simulink model "rsgTask_Complete_t5_bld"  (R2012b)
settings: Solver=FixedStepDiscrete  StartTime=0.0  StopTime=inf  FixedStep=0.001  RelTol=1e-3
settings Model: ExplicitPartitioning=on  Creator=gilja  LastModifiedBy=NPTL
settings SolverCC: EnableConcurrentExecution=on  ConcurrentTasks=on
settings OptimizationCC: InlineParams=on  InlineInvariantSignals=on  EnhancedBackFolding=on  EfficientFloat2IntCast=on
settings HardwareCC: ProdIntDivRoundTo=Zero  ProdEndianess=LittleEndian  ProdHWDeviceType=Generic->32-bit x86 compatible
settings ModelReferenceCC: UpdateModelReferenceTargets=IfOutOfDate  ModelReferenceMinAlgLoopOccurrences=on
settings RTWCC: SystemTargetFile=xpctarget.tlc  TLCOptions=-axPCMaxOverloads=10000 -axPCOverLoadLen=5 -axPCStartupFlag=200  TemplateMakefile=xpc_default_tmf  Description=xPC Target  ProcessScript=xpctarget_make_rtw_hook  RTWUseSimCustomCode=on  RTWCompilerOptimization=On
settings CodeAppCC: MaxIdLength=62
settings xpcTargetCC: TargetFcnLib=ansi_tfl_table_tmw.mat  CodeReplacementLibrary=XPC_BLAS  ParMdlRefBuildCompliant=on  ConcurrentExecutionCompliant=on  CombineSignalStateStructs=off  GRTInterface=on  xPCTaskExecutionProfile=on  xPCRL32EventNumber=5000  RL32IRQSourceModifier=5  xPCIRQSourceBoard=Parallel_Port  xPCIOIRQSlot=0x378  xPCisDownloadable=off  xPCLoadParamSetFile=off  xPCConcurrentTasks=off  xPCEnableSFAnimation=off

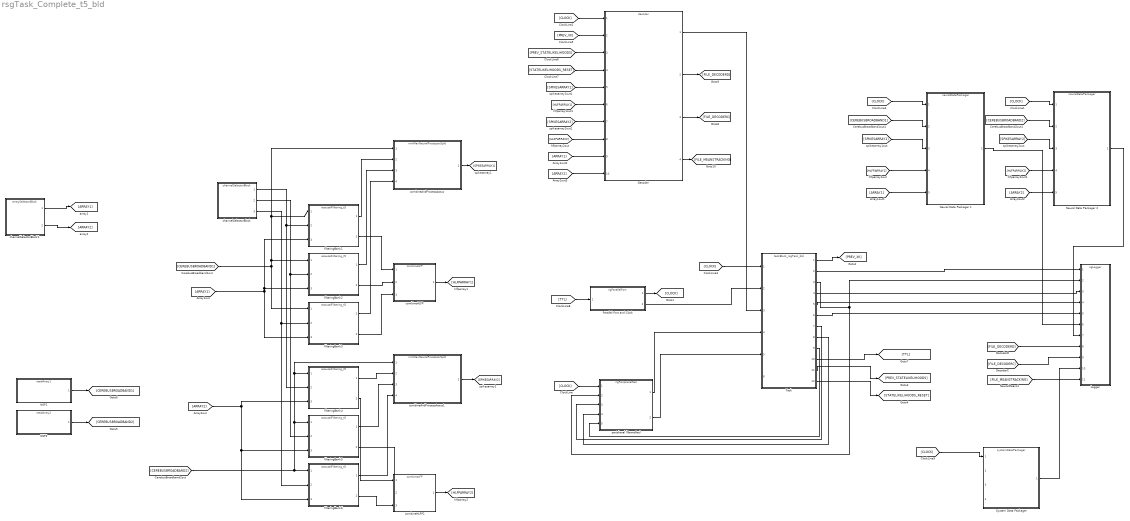
== system rsgTask_Complete_t5_bld ==
  Decoder : ModelReference  ModelNameDialog=decoder  SimulationMode=Normal  ModelReferenceVersion=1.1425  CopyOfModelName=decoder  DefaultDataLogging=on
  Logger : ModelReference  ModelNameDialog=rigLogger  SimulationMode=Normal  ModelReferenceVersion=1.138  CopyOfModelName=rigLogger  DefaultDataLogging=on
  NSP1 : ModelReference  ModelNameDialog=readArray1  SimulationMode=Normal  ModelReferenceVersion=1.166  CopyOfModelName=readArray1  DefaultDataLogging=on
  NSP2 : ModelReference  ModelNameDialog=readArray2  SimulationMode=Normal  ModelReferenceVersion=1.127  CopyOfModelName=readArray2  DefaultDataLogging=on
  Neural Data Packager 1 : ModelReference  ModelNameDialog=neuralDataPackager  SimulationMode=Normal  ModelReferenceVersion=1.174  CopyOfModelName=neuralDataPackager  DefaultDataLogging=on
  Neural Data Packager 2 : ModelReference  ModelNameDialog=neuralDataPackager  SimulationMode=Normal  ModelReferenceVersion=1.174  CopyOfModelName=neuralDataPackager  DefaultDataLogging=on
  Parallel Port and Clock : ModelReference  ModelNameDialog=rigParallelPort  SimulationMode=Normal  ModelReferenceVersion=1.93  CopyOfModelName=rigParallelPort  DefaultDataLogging=on
  System Data Packager : ModelReference  Priority=0  ModelNameDialog=systemDataPackager  SimulationMode=Normal  ModelReferenceVersion=1.180  CopyOfModelName=systemDataPackager  DefaultDataLogging=on
  Task : ModelReference  ModelNameDialog=taskBlock_rsgTask_bld  SimulationMode=Normal  ModelReferenceVersion=1.983  CopyOfModelName=taskBlock_rsgTask_bld  DefaultDataLogging=on
  channelSelectorBlock : ModelReference  ModelNameDialog=channelSelectorBlock  SimulationMode=Normal  ModelReferenceVersion=1.36  CopyOfModelName=channelSelectorBlock  DefaultDataLogging=on
  channelSelectorBlock1 : ModelReference  ModelNameDialog=arraySelectorBlock  SimulationMode=Normal  ModelReferenceVersion=1.40  CopyOfModelName=arraySelectorBlock  DefaultDataLogging=on
  combineAndProcessAcaus : ModelReference  ModelNameDialog=minMaxNeuralProcessorSplit  SimulationMode=Normal  ModelReferenceVersion=1.38  CopyOfModelName=minMaxNeuralProcessorSplit  DefaultDataLogging=on
  combineAndProcessAcaus1 : ModelReference  ModelNameDialog=minMaxNeuralProcessorSplit  SimulationMode=Normal  ModelReferenceVersion=1.38  CopyOfModelName=minMaxNeuralProcessorSplit  DefaultDataLogging=on
  combineHLFP : ModelReference  ModelNameDialog=combineLFP  SimulationMode=Normal  ModelReferenceVersion=1.38  CopyOfModelName=combineLFP  DefaultDataLogging=on
  combineHLFP1 : ModelReference  ModelNameDialog=combineLFP  SimulationMode=Normal  ModelReferenceVersion=1.38  CopyOfModelName=combineLFP  DefaultDataLogging=on
  filteringBank{1..6} (6 alike) : ModelReference  ModelNameDialog=acausalFiltering_t5  SimulationMode=Normal  ModelReferenceVersion=1.78  CopyOfModelName=acausalFiltering_t5  DefaultDataLogging=on
  peripheral (GameNet) : ModelReference  ModelNameDialog=rigPeripheralNet  SimulationMode=Normal  ModelReferenceVersion=1.372  CopyOfModelName=rigPeripheralNet  DefaultDataLogging=on
  wires:
  filteringBank1/1 -> combineAndProcessAcaus/2
  channelSelectorBlock/1 -> filteringBank4/2, filteringBank1/2
  channelSelectorBlock/2 -> filteringBank5/2, filteringBank2/2
  filteringBank2/1 -> combineAndProcessAcaus/3
  channelSelectorBlock/3 -> filteringBank6/2, filteringBank3/2
  filteringBank3/1 -> combineAndProcessAcaus/4
  filteringBank1/2 -> combineHLFP/1
  filteringBank2/2 -> combineHLFP/2
  filteringBank3/2 -> combineHLFP/3
  Parallel Port and Clock/2 -> Task/2
  [SPIKESARRAY1] -> Neural Data Packager 1/3
  Decoder/1 -> Task/3
  Neural Data Packager 1/1 -> Logger/6
  Task/2 -> Logger/1
  Task/3 -> peripheral (GameNet)/2, Logger/2
  Task/4 -> Logger/3
  Task/5 -> Logger/4
  Task/6 -> Logger/5
  Task/7 -> peripheral (GameNet)/3
  peripheral (GameNet)/1 -> Task/4
  peripheral (GameNet)/2 -> Task/5
  Task/9 -> peripheral (GameNet)/5
  Task/8 -> peripheral (GameNet)/4
  [CEREBUSBROADBAND1] -> filteringBank3/1, filteringBank2/1, combineAndProcessAcaus/1, filteringBank1/1
  [CEREBUSBROADBAND2] -> filteringBank6/1, filteringBank5/1, filteringBank4/1, combineAndProcessAcaus1/1
  filteringBank5/2 -> combineHLFP1/2
  filteringBank4/2 -> combineHLFP1/1
  filteringBank6/2 -> combineHLFP1/3
  filteringBank4/1 -> combineAndProcessAcaus1/2
  filteringBank5/1 -> combineAndProcessAcaus1/3
  filteringBank6/1 -> combineAndProcessAcaus1/4
  Neural Data Packager 2/1 -> Logger/7
  [ARRAY1] -> filteringBank3/3, filteringBank1/3, filteringBank2/3
  [ARRAY2] -> filteringBank4/3, filteringBank6/3, filteringBank5/3
  Parallel Port and Clock/1 -> [CLOCK]
  [CLOCK] -> peripheral (GameNet)/1
  [CLOCK] -> Neural Data Packager 2/1
  [CLOCK] -> Decoder/1
  [CLOCK] -> Task/1
  [CLOCK] -> Neural Data Packager 1/1
  combineHLFP/1 -> [HLFPARRAY1]
  [HLFPARRAY1] -> Neural Data Packager 1/4
  [HLFPARRAY1] -> Decoder/6
  combineHLFP1/1 -> [HLFPARRAY2]
  [HLFPARRAY2] -> Decoder/8
  [HLFPARRAY2] -> Neural Data Packager 2/4
  combineAndProcessAcaus1/1 -> [SPIKESARRAY2]
  [SPIKESARRAY2] -> Neural Data Packager 2/3
  [SPIKESARRAY2] -> Decoder/7
  combineAndProcessAcaus/1 -> [SPIKESARRAY1]
  [SPIKESARRAY1] -> Decoder/5
  Task/1 -> [PREV_XK]
  [PREV_XK] -> Decoder/2
  Task/11 -> [PREV_STATELIKELIHOODS]
  [PREV_STATELIKELIHOODS] -> Decoder/3
  Task/12 -> [STATELIKELIHOODS_RESET]
  [STATELIKELIHOODS_RESET] -> Decoder/4
  [CEREBUSBROADBAND1] -> Neural Data Packager 1/2
  [CEREBUSBROADBAND2] -> Neural Data Packager 2/2
  channelSelectorBlock1/1 -> [ARRAY1]
  channelSelectorBlock1/2 -> [ARRAY2]
  [ARRAY2] -> Neural Data Packager 2/5
  [ARRAY1] -> Neural Data Packager 1/5
  [ARRAY1] -> Decoder/9
  [ARRAY2] -> Decoder/10
  NSP1/1 -> [CEREBUSBROADBAND1]
  Task/10 -> [TTL]
  [TTL] -> Parallel Port and Clock/1
  NSP2/1 -> [CEREBUSBROADBAND2]
  [CLOCK] -> System Data Packager/1
  System Data Packager/1 -> Logger/10
  Decoder/2 -> [FILE_DECODERD]
  Decoder/3 -> [FILE_DECODERC]
  [FILE_DECODERD] -> Logger/8
  [FILE_DECODERC] -> Logger/9
  Decoder/4 -> [FILE_MEANSTRACKING]
  [FILE_MEANSTRACKING] -> Logger/11
  ? -> System Data Packager/2
  ? -> System Data Packager/3
  ? -> System Data Packager/4
